simulink model "Project_Task2_4328802_SinghShrestha"  (Simulink 8.0)
settings: Solver=ode45  StartTime=0.0  StopTime=80*Ts  RelTol=1e-3
PreLoadFcn:
  | Ts=20e-9; % Sample period
  | W=6;        % Bit-width
  | 
  | x_constant = 12;
  | gap = 100;
  | 
  | % Input sequence for x signal
  | x_value = [0 x_constant zeros(1,gap)]';   %value
  | x_time = [0:length(x_value)-1]'*Ts;          % time
  | x = [x_time x_value];                              % signal
  | 
  | % Input sequence for start signal
  | start_value = [0 1 zeros(1,gap)]';   % value
  | start_time = [0:length(start_value)-1]'*Ts;  % time
  | start = [start_time start_value];                 % signal
undefined symbols (not defined in the file): xlipgetpartsetting
libraries: xbsIndex_r4 x51
settings Model: Creator=alpha  LastModifiedBy=SaGuN MS
settings DataIOCC: SignalLoggingSaveFormat=ModelDataLogs
settings OptimizationCC: InitFltsAndDblsToZero=on
settings DebuggingCC: SaveWithParameterizedLinksMsg=none  SignalResolutionControl=TryResolveAllWithWarning  MultiTaskDSMMsg=warning  MultiTaskCondExecSysMsg=none  FcnCallInpInsideContextMsg=UseLocalSettings  StrictBusMsg=Warning
settings RTWCC: IncludeERTFirstTime=on
settings GRTTargetCC: TargetFcnLib=ansi_tfl_tmw.mat  CombineOutputUpdateFcns=off  GRTInterface=on

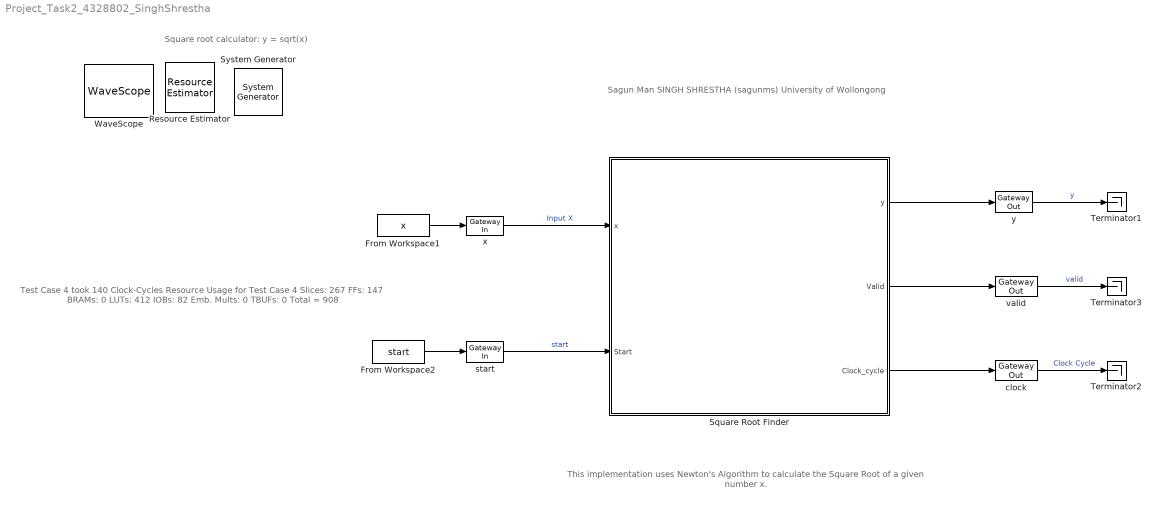
== system Project_Task2_4328802_SinghShrestha ==
  note: Square root calculator: y = sqrt(x)
  note: Sagun Man SINGH SHRESTHA
      | (sagunms)
      | University of Wollongong
  note: Test Case 4 took 140 Clock-Cycles
      |
      | Resource Usage for Test Case 4
      | Slices: 267
      | FFs: 147
      | BRAMs: 0
      | LUTs: 412
      | IOBs: 82
      | Emb. Mults: 0
      | TBUFs: 0
      | Total = 908
  note: This implementation uses Newton's Algorithm to calculate the Square Root of a given number x.
  " System Generator" : xbsIndex_r4/ System Generator  Tag=genX  xilinxfamily=spartan3e  part=xc3s500e  speed=-4  package=fg320  synthesis_tool=XST  clock_wrapper=Clock Enables  directory=./ise  proj_type=Project Navigator  Synth_file=XST Defaults  Impl_file=ISE Defaults  testbench=off  simulink_period=Ts  sysclk_period=20  dcm_input_clock_period=100  incr_netlist=off  trim_vbits=Everywhere in SubSystem  dbl_ovrd=According to Block Masks  core_generation=According to Block Masks  run_coregen=off  deprecated_control=off  eval_field=0  block_type=sysgen
      settings: block_version=8.2.02
  From Workspace1 : FromWorkspace  VariableName=x  SampleTime=Ts  Interpolate=off  OutputAfterFinalValue=Holding final value
  From Workspace2 : FromWorkspace  VariableName=start  SampleTime=Ts  Interpolate=off  OutputAfterFinalValue=Holding final value
  Resource Estimator : xbsIndex_r4/Resource Estimator  Tag=resEstTag  Slices=267  FFs=147  BRAMs=0  LUTs=412  IOBs=82  EBMs=0  TBUFs=0  xl_use_estimator_area=off  est_options=Estimate  xl_estimator_area="[ 267  147    0  412   82    0    0 ]"  block_type=resource_estimator
      settings: AttributesFormatString=Resource\nEstimator  block_version=11.4
  Square Root Finder : Subsystem
  Terminator1 : Terminator
  Terminator2 : Terminator
  Terminator3 : Terminator
  WaveScope : xbsIndex_r4/WaveScope  block_type=wavescope
      settings: block_version=8.2.02
  clock : xbsIndex_r4/Gateway Out  inherit_from_input=off  hdl_port=on  timing_constraint=None  locs_specified=off  LOCs={'F9'}  UseAsDAC=off  DACChannel='1'  block_type=gatewayout
      settings: infoedit="Gateway out block.  Converts Xilinx fixed point inputs into ouputs of type Simulink integer, double, or fixed point.<P><P>Hardware notes:  In hardware these blocks become top level output ports or are discarded, depending on how they are configured."  xl_area=[0 0 0 0 40 0 0]  block_version=8.2.02
  start : xbsIndex_r4/Gateway In  gui_display_data_type=Fixed-point  arith_type=Boolean  n_bits=W  bin_pt=0  preci_type=Single  exp_width=8  frac_width=24  quantization="Round  (unbiased: +/- Inf)"  overflow=Wrap  period=Ts  dbl_ovrd=off  timing_constraint=None  locs_specified=off  LOCs={'V16'}  UseAsADC=off  ADCChannel='1'  inherit_from_input=off  hdl_port=on  block_type=gatewayin
      settings: infoedit="Gateway in block.  Converts inputs of type Simulink integer, double and fixed point to  Xilinx fixed point type.<P><P>Hardware notes:  In hardware these blocks become top level input ports."  xl_area=[0 0 0 0 1 0 0]  block_version=8.2.02
  valid : xbsIndex_r4/Gateway Out  inherit_from_input=off  hdl_port=on  timing_constraint=None  locs_specified=off  LOCs={'F9'}  UseAsDAC=off  DACChannel='1'  block_type=gatewayout
      settings: infoedit="Gateway out block.  Converts Xilinx fixed point inputs into ouputs of type Simulink integer, double, or fixed point.<P><P>Hardware notes:  In hardware these blocks become top level output ports or are discarded, depending on how they are configured."  xl_area=[0 0 0 0 1 0 0]  block_version=8.2.02
  x : xbsIndex_r4/Gateway In  gui_display_data_type=Fixed-point  arith_type=Unsigned  n_bits=W  bin_pt=0  preci_type=Single  exp_width=8  frac_width=24  quantization="Round  (unbiased: +/- Inf)"  overflow=Wrap  period=Ts  dbl_ovrd=off  timing_constraint=None  locs_specified=off  LOCs={'V16'}  UseAsADC=off  ADCChannel='1'  inherit_from_input=off  hdl_port=on  block_type=gatewayin
      settings: infoedit="Gateway in block.  Converts inputs of type Simulink integer, double and fixed point to  Xilinx fixed point type.<br><br>Hardware notes:  In hardware these blocks become top level input ports."  xl_area=[0 0 0 0 20 0 0]  block_version=8.2.02
  y : xbsIndex_r4/Gateway Out  inherit_from_input=off  hdl_port=on  timing_constraint=None  locs_specified=off  LOCs={'F9'}  UseAsDAC=off  DACChannel='1'  block_type=gatewayout
      settings: infoedit="Gateway out block.  Converts Xilinx fixed point inputs into ouputs of type Simulink integer, double, or fixed point.<P><P>Hardware notes:  In hardware these blocks become top level output ports or are discarded, depending on how they are configured."  xl_area=[0 0 0 0 20 0 0]  block_version=8.2.02
  wires:
  From Workspace1/1 -> x/1
  From Workspace2/1 -> start/1
  clock/1 -> Terminator2/1  "Clock Cycle"
  x/1 -> Square Root Finder/1(x)  "Input X"
  start/1 -> Square Root Finder/2(Start)  "start"
  Square Root Finder/1(y) -> y/1
  Square Root Finder/2(Valid) -> valid/1
  Square Root Finder/3(Clock_cycle) -> clock/1
  y/1 -> Terminator1/1  "y"
  valid/1 -> Terminator3/1  "valid"

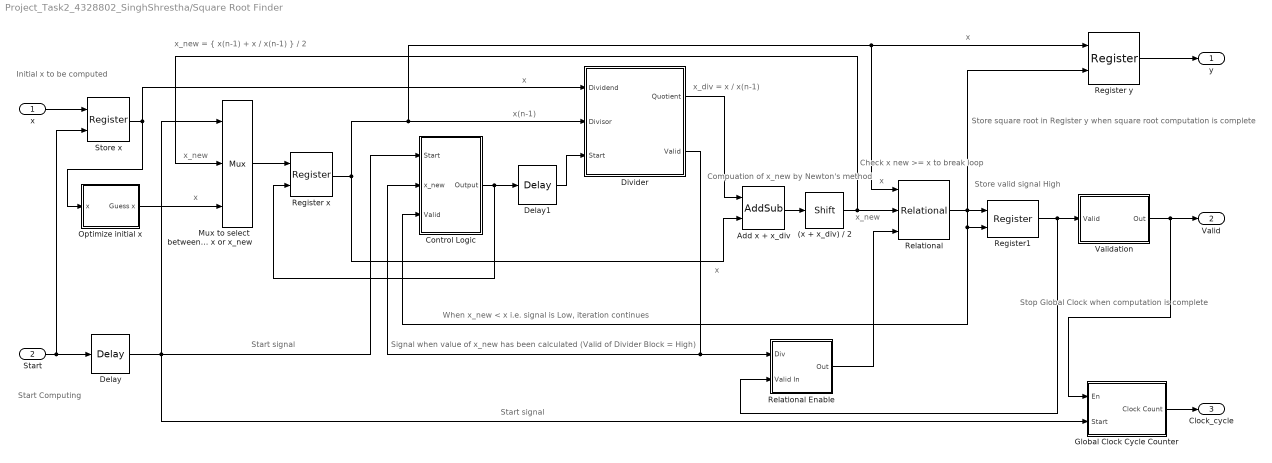
== system Project_Task2_4328802_SinghShrestha/Square Root Finder ==
  note: When x_new < x i.e. signal is Low, iteration continues
  note: x
  note: x_div = x / x(n-1)
  note: x_new = { x(n-1) + x / x(n-1) } / 2
  note: x
  note: Check x new >= x
      | to break loop
  note: x_new
  note: x
  note: Store valid signal High
  note: x
  note: Start Computing
  note: x(n-1)
  note: x_new
  note: Initial x to be computed
  note: Store square root in Register y
      | when square root computation
      | is complete
  note: Start signal
  note: x
  note: Start signal
  note: Signal when value of x_new has been calculated (Valid of Divider Block = High)
  note: Compuation of x_new by
      | Newton's method
  note: Stop Global Clock when
      | computation is complete
  x : Inport
  Start : Inport  Port=2
  (x + x_div) / 2 : xbsIndex_r4/Shift  shift_dir=Right  shift_bits=1  en=off  latency=0  precision=Full  arith_type="Signed  (2's comp)"  n_bits=16  bin_pt=14  quantization=Truncate  overflow=Wrap  dbl_ovrd=off  block_type=shift
      settings: xl_area=[0 0 0 0 0 0 0]
  Add x + x_div : xbsIndex_r4/AddSub  mode=Addition  use_carryin=off  use_carryout=off  en=off  latency=0  precision=User Defined  arith_type=Unsigned  n_bits=W  bin_pt=0  quantization=Truncate  overflow=Wrap  dbl_ovrd=off  use_behavioral_HDL=off  hw_selection=Fabric  pipelined=off  use_rpm=on  block_type=addsub
      settings: xl_area=[10 0 0 20 0 0 0]  block_version=8.2.02
  Control Logic : Subsystem
  Delay : xbsIndex_r4/Delay  rst=off  infoeditControl=Selection of Reset will increase slice count due to use of real FFs and instead of SRLs  en=off  latency=1  dbl_ovrd=off  reg_retiming=off  block_type=delay
      settings: infoedit=Hardware notes: A delay line is a chain, each link of which is an SRL16 followed by a flip-flop. If register retiming is enabled, the delay line is a chain of flip-flops.  xl_area=[1 1 0 0 0 0 0]  block_version=8.2.02
  Delay1 : xbsIndex_r4/Delay  rst=off  infoeditControl=Selection of Reset will increase slice count due to use of real FFs and instead of SRLs  en=off  latency=1  dbl_ovrd=off  reg_retiming=off  block_type=delay
      settings: infoedit=Hardware notes: A delay line is a chain, each link of which is an SRL16 followed by a flip-flop. If register retiming is enabled, the delay line is a chain of flip-flops.  xl_area=[1 1 0 0 0 0 0]  block_version=8.2.02
  Divider : Subsystem
  Global Clock Cycle Counter : Subsystem
  Mux to select  between x or x_new : xbsIndex_r4/Mux  inputs=2  en=off  latency=0  precision=Full  arith_type=Unsigned  n_bits=16  bin_pt=14  quantization=Truncate  overflow=Wrap  dbl_ovrd=off  block_type=mux
      settings: xl_area=[10 0 0 20 0 0 0]  block_version=8.2.02
  Optimize initial x : Subsystem
  Register x : xbsIndex_r4/Register  init=0  rst=off  en=on  dbl_ovrd=off  block_type=register
      settings: xl_area=[10 20 0 0 0 0 0]  block_version=8.2.02
  Register y : xbsIndex_r4/Register  init=0  rst=off  en=on  dbl_ovrd=off  block_type=register
      settings: xl_area=[10 20 0 0 0 0 0]  block_version=11.4
  Register1 : xbsIndex_r4/Register  init=0  rst=off  en=on  dbl_ovrd=off  block_type=register
      settings: xl_area=[1 1 0 0 0 0 0]  block_version=11.4
  Relational : xbsIndex_r4/Relational  mode=a<=b  en=on  latency=1  dbl_ovrd=off  block_type=relational
      settings: xl_area=[11 1 0 21 0 0 0]  block_version=8.2.02
  Relational Enable : Subsystem
  Store x : xbsIndex_r4/Register  init=0  rst=off  en=on  dbl_ovrd=off  block_type=register
      settings: xl_area=[10 20 0 0 0 0 0]  block_version=8.2.02
  Validation : Subsystem
  y : Outport
  Valid : Outport  Port=2
  Clock_cycle : Outport  Port=3
  wires:
  Store x/1 -> Optimize initial x/1(x), Divider/1(Dividend)
  Start/1 -> Delay/1, Store x/2
  Delay/1 -> Global Clock Cycle Counter/2(Start), Control Logic/1(Start), Mux to select  between x or x_new/1
  Mux to select  between x or x_new/1 -> Register x/1
  Register x/1 -> Add x + x_div/2, Divider/2(Divisor), Register y/1, Relational/1
  Register1/1 -> Relational Enable/2(Valid In), Validation/1(Valid)
  Relational/1 -> Control Logic/3(Valid), Register1/2, Register y/2, Register1/1
  Control Logic/1(Output) -> Delay1/1, Register x/2
  Divider/1(Quotient) -> Add x + x_div/1
  Delay1/1 -> Divider/3(Start)
  Relational Enable/1(Out) -> Relational/3
  Validation/1(Out) -> Valid/1, Global Clock Cycle Counter/1(En)
  Register y/1 -> y/1
  x/1 -> Store x/1
  Global Clock Cycle Counter/1(Clock Count) -> Clock_cycle/1
  Optimize initial x/1(Guess x) -> Mux to select  between x or x_new/3
  Add x + x_div/1 -> (x + x_div) / 2/1
  (x + x_div) / 2/1 -> Relational/2, Mux to select  between x or x_new/2
  Divider/2(Valid) -> Control Logic/2(x_new), Relational Enable/1(Div)

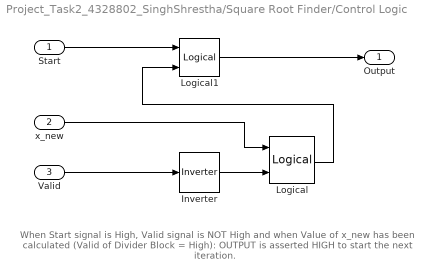
== system Project_Task2_4328802_SinghShrestha/Square Root Finder/Control Logic ==
  note: When Start signal is High, Valid signal is NOT High
      | and when Value of x_new has been calculated (Valid of Divider Block = High):
      | OUTPUT is asserted HIGH to start the next iteration.
  Start : Inport
  x_new : Inport  Port=2
  Valid : Inport  Port=3
  Inverter : xbsIndex_r4/Inverter  en=off  latency=0  dbl_ovrd=off  block_type=inv
      settings: xl_area=[0 0 0 0 0 0 0]  block_version=11.4
  Logical : xbsIndex_r4/Logical  logical_function=AND  inputs=2  en=off  latency=0  precision=Full  arith_type=Unsigned  n_bits=16  bin_pt=0  align_bp=on  dbl_ovrd=off  block_type=logical
      settings: xl_area=[1 0 0 1 0 0 0]  block_version=11.4
  Logical1 : xbsIndex_r4/Logical  logical_function=OR  inputs=2  en=off  latency=0  precision=Full  arith_type=Unsigned  n_bits=16  bin_pt=0  align_bp=on  dbl_ovrd=off  block_type=logical
      settings: xl_area=[1 0 0 1 0 0 0]  block_version=11.4
  Output : Outport
  wires:
  Logical/1 -> Logical1/2
  Valid/1 -> Inverter/1
  Logical1/1 -> Output/1
  Inverter/1 -> Logical/2
  x_new/1 -> Logical/1
  Start/1 -> Logical1/1

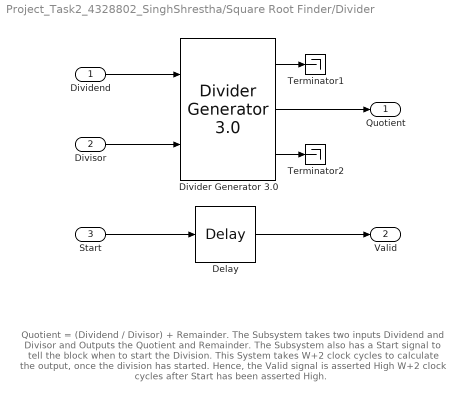
== system Project_Task2_4328802_SinghShrestha/Square Root Finder/Divider ==
  note: Quotient = (Dividend / Divisor) + Remainder.
      |
      | The Subsystem takes two inputs Dividend and Divisor and Outputs the Quotient and Remainder.
      | The Subsystem also has a Start signal to tell the block when to start the Division.
      |
      | This System takes W+2 clock cycles to calculate the output, once the division has started.
      | Hence, the Valid signal is asserted High W+2 clock cycles after Start has been asserted High.
  Dividend : Inport
  Divisor : Inport  Port=2
  Start : Inport  Port=3
  Delay : xbsIndex_r4/Delay  rst=off  infoeditControl=Selection of Reset will increase slice count due to use of real FFs and instead of SRLs  en=off  latency=W+2  dbl_ovrd=off  reg_retiming=off  block_type=delay
      settings: xl_area=[2 2 0 2 0 0 0]  block_version=11.4
  "Divider Generator 3.0 " : xbsIndex_r4/Divider Generator 3.0   dividend_and_quotient_width=W  divisor_width=W  algorithm_type=Radix2  remainder_type=Remainder  fractional_width=16  clocks_per_division=1  divide_by_zero_detect=off  latency_configuration=Automatic  latency=20  ce=off  sclr=off  sclr_ce_priority=SCLR_overrides_CE  operand_sign=Signed  ip_name=Divider Generator  ip_version=3.0  dsptool_ready=true  wrapper_available=true  port_translation_map={ 'ce' => 'en', 'sclr' => 'rst' }  ipcore_fpga_part=xlipgetpartsetting(gcb, {'virtex4', 'xc4vsx35', '-10', 'ff668'})  ipcore_verbose=false  block_type=div_gen_v3_0
      settings: xl_area=[672 1282 0 439 0 0 0]  block_version=11.4
  Terminator1 : Terminator
  Terminator2 : Terminator
  Quotient : Outport
  Valid : Outport  Port=2
  wires:
  "Divider Generator 3.0 "/1 -> Terminator1/1
  Dividend/1 -> "Divider Generator 3.0 "/1
  "Divider Generator 3.0 "/2 -> Quotient/1
  Divisor/1 -> "Divider Generator 3.0 "/2
  "Divider Generator 3.0 "/3 -> Terminator2/1
  Start/1 -> Delay/1
  Delay/1 -> Valid/1

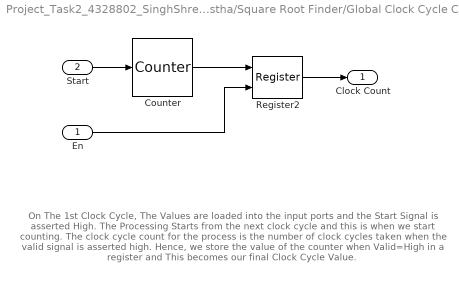
== system Project_Task2_4328802_SinghShrestha/Square Root Finder/Global Clock Cycle Counter ==
  note: On The 1st Clock Cycle, The Values are loaded into the input ports and the Start Signal is asserted High.
      |
      | The Processing Starts from the next clock cycle and this is when we start counting.
      | The clock cycle count for the process is the number of clock cycles taken when the valid signal is asserted high.
      |
      | Hence, we store the value of the counter when Valid=High in a register and This becomes our final Clock Cycle Value.
  En : Inport
  Start : Inport  Port=2
  Counter : xbsIndex_r4/Counter  cnt_type=Free Running  cnt_to=Inf  operation=Up  start_count=1  cnt_by_val=1  arith_type=Unsigned  n_bits=2*W  bin_pt=0  load_pin=off  rst=on  en=off  explicit_period=off  period=1  dbl_ovrd=off  use_behavioral_HDL=off  implementation=Fabric  use_rpm=off  block_type=counter
      settings: xl_area=[21 40 0 40 0 0 0]  block_version=8.2.02
  Register2 : xbsIndex_r4/Register  init=0  rst=off  en=on  dbl_ovrd=off  block_type=register
      settings: xl_area=[20 40 0 0 0 0 0]  block_version=11.4
  Clock Count : Outport
  wires:
  Counter/1 -> Register2/1
  Register2/1 -> Clock Count/1
  Start/1 -> Counter/1
  En/1 -> Register2/2

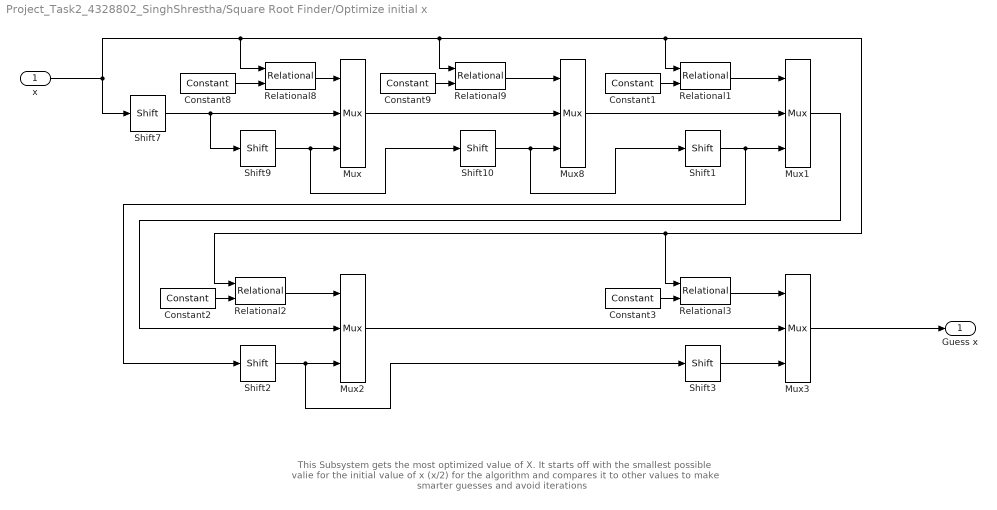
== system Project_Task2_4328802_SinghShrestha/Square Root Finder/Optimize initial x ==
  note: This Subsystem gets the most optimized value of X.
      | It starts off with the smallest possible valie for the initial value of x (x/2) for
      | the algorithm and compares it to other values to make smarter guesses and avoid iterations
  x : Inport
  Constant1 : xbsIndex_r4/Constant  const=256  gui_display_data_type=Fixed-point  arith_type=Unsigned  n_bits=2*W  bin_pt=0  preci_type=Single  exp_width=8  frac_width=24  explicit_period=on  period=1  equ=P=C  opselect=C  inp2=PCIN>>17  opr=+  inp1=P  carry=CIN  dbl_ovrd=off  block_type=constant
      settings: block_version=11.4
  Constant2 : xbsIndex_r4/Constant  const=1024  gui_display_data_type=Fixed-point  arith_type=Unsigned  n_bits=2*W  bin_pt=0  preci_type=Single  exp_width=8  frac_width=24  explicit_period=on  period=1  equ=P=C  opselect=C  inp2=PCIN>>17  opr=+  inp1=P  carry=CIN  dbl_ovrd=off  block_type=constant
      settings: block_version=11.4
  Constant3 : xbsIndex_r4/Constant  const=4096  gui_display_data_type=Fixed-point  arith_type=Unsigned  n_bits=2*W  bin_pt=0  preci_type=Single  exp_width=8  frac_width=24  explicit_period=on  period=1  equ=P=C  opselect=C  inp2=PCIN>>17  opr=+  inp1=P  carry=CIN  dbl_ovrd=off  block_type=constant
      settings: block_version=11.4
  Constant8 : xbsIndex_r4/Constant  const=16  gui_display_data_type=Fixed-point  arith_type=Unsigned  n_bits=2*W  bin_pt=0  preci_type=Single  exp_width=8  frac_width=24  explicit_period=on  period=1  equ=P=C  opselect=C  inp2=PCIN>>17  opr=+  inp1=P  carry=CIN  dbl_ovrd=off  block_type=constant
      settings: block_version=11.4
  Constant9 : xbsIndex_r4/Constant  const=64  gui_display_data_type=Fixed-point  arith_type=Unsigned  n_bits=2*W  bin_pt=0  preci_type=Single  exp_width=8  frac_width=24  explicit_period=on  period=1  equ=P=C  opselect=C  inp2=PCIN>>17  opr=+  inp1=P  carry=CIN  dbl_ovrd=off  block_type=constant
      settings: block_version=11.4
  Mux{,1..3,8} (5 alike) : xbsIndex_r4/Mux  inputs=2  en=off  latency=0  precision=Full  arith_type=Unsigned  n_bits=16  bin_pt=14  quantization=Truncate  overflow=Wrap  dbl_ovrd=off  block_type=mux
      settings: xl_area=[10 0 0 20 0 0 0]  block_version=11.4
  Relational{1..3,8..9} (5 alike) : xbsIndex_r4/Relational  mode=a>=b  en=off  latency=0  dbl_ovrd=off  block_type=relational
      settings: xl_area=[21 0 0 41 0 0 0]  block_version=8.2.02
  Shift{1..3,7,9..10} (6 alike) : xbsIndex_r4/Shift  shift_dir=Right  shift_bits=1  en=off  latency=0  precision=Full  arith_type="Signed  (2's comp)"  n_bits=W  bin_pt=0  quantization=Truncate  overflow=Wrap  dbl_ovrd=off  block_type=shift
      settings: xl_area=[0 0 0 0 0 0 0]
  Guess x : Outport
  wires:
  Relational8/1 -> Mux/1
  Constant8/1 -> Relational8/2
  Mux/1 -> Mux8/2
  Relational9/1 -> Mux8/1
  Constant9/1 -> Relational9/2
  Shift7/1 -> Mux/2, Shift9/1
  Shift9/1 -> Mux/3, Shift10/1
  Shift10/1 -> Mux8/3, Shift1/1
  Mux8/1 -> Mux1/2
  Relational1/1 -> Mux1/1
  Constant1/1 -> Relational1/2
  Shift1/1 -> Mux1/3, Shift2/1
  Mux1/1 -> Mux2/2
  Relational2/1 -> Mux2/1
  Constant2/1 -> Relational2/2
  Shift2/1 -> Mux2/3, Shift3/1
  Mux2/1 -> Mux3/2
  Relational3/1 -> Mux3/1
  Constant3/1 -> Relational3/2
  Shift3/1 -> Mux3/3
  Mux3/1 -> Guess x/1
  x/1 -> Relational2/1, Relational3/1, Relational1/1, Relational9/1, Relational8/1, Shift7/1

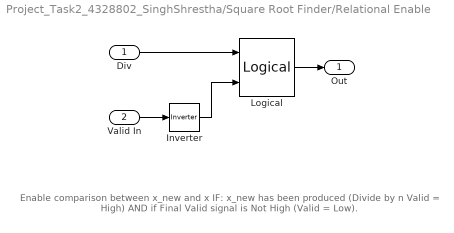
== system Project_Task2_4328802_SinghShrestha/Square Root Finder/Relational Enable ==
  note: Enable comparison between x_new and x IF:
      |  x_new has been produced (Divide by n Valid = High)
      | AND
      | if Final Valid signal is Not High (Valid = Low).
  Div : Inport
  Valid In : Inport  Port=2
  Inverter : xbsIndex_r4/Inverter  en=off  latency=0  dbl_ovrd=off  block_type=inv
      settings: xl_area=[0 0 0 0 0 0 0]  block_version=11.4
  Logical : xbsIndex_r4/Logical  logical_function=AND  inputs=2  en=off  latency=0  precision=Full  arith_type=Unsigned  n_bits=16  bin_pt=0  align_bp=on  dbl_ovrd=off  block_type=logical
      settings: xl_area=[1 0 0 1 0 0 0]  block_version=11.4
  Out : Outport
  wires:
  Inverter/1 -> Logical/2
  Div/1 -> Logical/1
  Logical/1 -> Out/1
  Valid In/1 -> Inverter/1

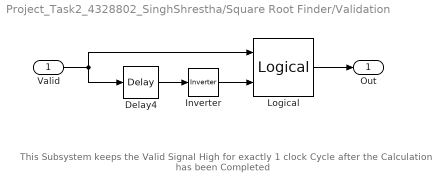
== system Project_Task2_4328802_SinghShrestha/Square Root Finder/Validation ==
  note: This Subsystem keeps the Valid Signal High for exactly 1 clock Cycle
      |  after the Calculation has been Completed
  Valid : Inport
  Delay4 : xbsIndex_r4/Delay  rst=off  infoeditControl=Selection of Reset will increase slice count due to use of real FFs and instead of SRLs  en=off  latency=1  dbl_ovrd=off  reg_retiming=off  block_type=delay
      settings: infoedit=Hardware notes: A delay line is a chain, each link of which is an SRL16 followed by a flip-flop. If register retiming is enabled, the delay line is a chain of flip-flops.  xl_area=[1 1 0 0 0 0 0]  block_version=8.2.02
  Inverter : xbsIndex_r4/Inverter  en=off  latency=0  dbl_ovrd=off  block_type=inv
      settings: xl_area=[0 0 0 0 0 0 0]  block_version=11.4
  Logical : xbsIndex_r4/Logical  logical_function=AND  inputs=2  en=off  latency=0  precision=Full  arith_type=Unsigned  n_bits=16  bin_pt=0  align_bp=on  dbl_ovrd=off  block_type=logical
      settings: xl_area=[1 0 0 1 0 0 0]  block_version=11.4
  Out : Outport
  wires:
  Inverter/1 -> Logical/2
  Delay4/1 -> Inverter/1
  Valid/1 -> Delay4/1, Logical/1
  Logical/1 -> Out/1
